simulink model "NeuromuscularModel_3R60_3D"  (R2019b)
settings: Solver=ode15s  StartTime=0.0  StopTime=30  MaxStep=.01  RelTol=1e-4  AbsTol=1e-6  EnableMultiTasking=on
values from neighbouring files (symbols this model uses):
  animFrameRate = 30    [demorun.m]    (also in optimize.m; optimizeCMG.m)
  dt_visual = 1/1000    (= 0.001)    [demorun.m]    (also in evaluateCost.m = 0.0333333333333; optimize.m = 0.0333333333333; optimizeCMG.m = 0.0333333333333; optimize_Conly.m = 0.0333333333333)
  initialTargetAngle = 70*pi/180    (= 1.2217304764)    [setInit.m]
  LPreStimBFSHinit = initConditionsSagittal(12)    [assignInit.m]
  LPreStimGASinit = initConditionsSagittal(13)    [assignInit.m]
  LPreStimGLUinit = initConditionsSagittal(8)    [assignInit.m]
  LPreStimHABinit = initConditionsCoronal(6)    [assignInit.m]
  LPreStimHADinit = initConditionsCoronal(7)    [assignInit.m]
  LPreStimHAMinit = initConditionsSagittal(9)    [assignInit.m]
  LPreStimHFLinit = initConditionsSagittal(7)    [assignInit.m]
  LPreStimRFinit = initConditionsSagittal(10)    [assignInit.m]
  LPreStimSOLinit = initConditionsSagittal(14)    [assignInit.m]
  LPreStimTAinit = initConditionsSagittal(15)    [assignInit.m]
  LPreStimVASinit = initConditionsSagittal(11)    [assignInit.m]
  LTargetAngleInit = initConditionsSagittal(6)    [assignInit.m]
  LTargetAngleRInit = initConditionsCoronal(5)    [assignInit.m]
  N = 133    [vcmaes_1.5cm_0.9ms_Umb10_kneelim1_mstoptorque2.mat]
  RPreStimGLUinit = initConditionsSagittal(18)    [assignInit.m]
  RPreStimHABinit = initConditionsCoronal(9)    [assignInit.m]
  RPreStimHADinit = initConditionsCoronal(10)    [assignInit.m]
  RPreStimHAMinit = initConditionsSagittal(19)    [assignInit.m]
  RPreStimHFLinit = initConditionsSagittal(17)    [assignInit.m]
  RPreStimRFinit = initConditionsSagittal(20)    [assignInit.m]
  RTargetAngleInit = initConditionsSagittal(16)    [assignInit.m]
  RTargetAngleRInit = initConditionsCoronal(8)    [assignInit.m]
undefined symbols (not defined in the file or in its folder): g, GaitState, hatLeftHipToCenterDistWidth, LongDelay, LongLoopDelay, MidDelay, ShortDelay, termination_height, thetaHATref, X, Y, Z
libraries: NeuroMuscularLibrary x105, nesl_utility x22, sm_lib x21, simulink x3, CMGlibrary x1
(part 2 of 3)

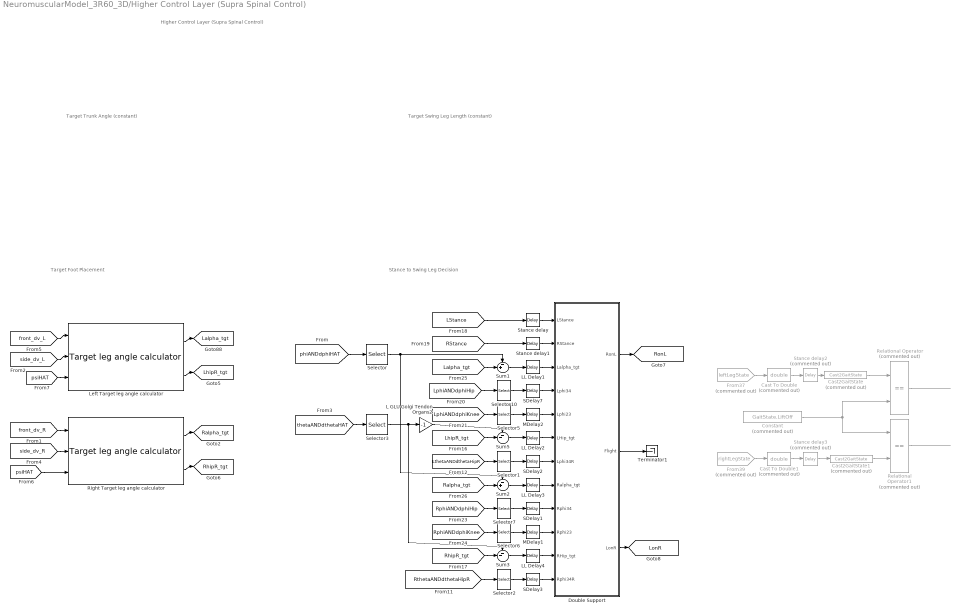
== system NeuromuscularModel_3R60_3D/Higher Control Layer (Supra Spinal Control) ==
  note: Target Foot Placement
  note: Target Swing Leg Length
      | (constant)
  note: Stance to Swing Leg Decision
  note: Target Trunk Angle
      | (constant)
  note: Higher Control Layer
      | (Supra Spinal Control)
  Cast To Double : DataTypeConversion  Commented=on  OutDataTypeStr=double
  Cast To Double1 : DataTypeConversion  Commented=on  OutDataTypeStr=double
  Cast2GaitState : NeuroMuscularLibrary/Cast2GaitState  Commented=on  SystemSampleTime=-1  Latency=0  AutoFrameSizeCalculation=off
  Cast2GaitState1 : NeuroMuscularLibrary/Cast2GaitState  Commented=on  SystemSampleTime=-1  Latency=0  AutoFrameSizeCalculation=off
  Constant : Constant  Commented=on  Value=GaitState.LiftOff
  Double Support : Subsystem
  From37 : From  Commented=on  GotoTag=leftLegState  TagVisibility=global
  From39 : From  Commented=on  GotoTag=rightLegState  TagVisibility=global
  L GLU Golgi Tendon Organs2 : Gain  Gain=-1
  LL Delay1 : TransportDelay  DelayTime=LongLoopDelay/2  InitialOutput=initialTargetAngle
  LL Delay2 : TransportDelay  DelayTime=LongLoopDelay/2
  LL Delay3 : TransportDelay  DelayTime=LongLoopDelay/2  InitialOutput=initialTargetAngle
  LL Delay4 : TransportDelay  DelayTime=LongLoopDelay/2
  Left Target leg angle calculator : NeuroMuscularLibrary/Target leg angle calculator  simbiconLegAngle0=LsimbiconLegAngle0  simbiconGainD=LsimbiconGainD  simbiconGainV=LsimbiconGainV  simbiconLegAngle0_C=LsimbiconLegAngle0_C  simbiconGainD_C=LsimbiconGainD_C  simbiconGainV_C=LsimbiconGainV_C  headingGain=LheadingGain
  MDelay1 : TransportDelay  DelayTime=MidDelay
  MDelay2 : TransportDelay  DelayTime=MidDelay
  Relational Operator : RelationalOperator  Commented=on  Operator===  OutDataTypeStr=boolean  RndMeth=Simplest
  Relational Operator1 : RelationalOperator  Commented=on  Operator===  OutDataTypeStr=boolean  RndMeth=Simplest
  Right Target leg angle calculator : NeuroMuscularLibrary/Target leg angle calculator  simbiconLegAngle0=RsimbiconLegAngle0  simbiconGainD=RsimbiconGainD  simbiconGainV=RsimbiconGainV  simbiconLegAngle0_C=RsimbiconLegAngle0_C  simbiconGainD_C=RsimbiconGainD_C  simbiconGainV_C=RsimbiconGainV_C  headingGain=RheadingGain
  SDelay{1..3,7} (4 alike) : TransportDelay  DelayTime=ShortDelay
  Selector : Selector  InputPortWidth=2  IndexOptions=Index vector (dialog)  Indices=[1]  OutputSizes=1
  Selector{1..2,5..7,10} (6 alike) : Selector  InputPortWidth=2  IndexOptions=Index vector (dialog)  Indices=1  OutputSizes=1
  Selector3 : Selector  InputPortWidth=2  IndexOptions=Index vector (dialog)  Indices=[1]  OutputSizes=1
  Stance delay : TransportDelay  DelayTime=MidDelay
  Stance delay1 : TransportDelay  DelayTime=MidDelay
  Stance delay2 : TransportDelay  Commented=on  DelayTime=MidDelay
  Stance delay3 : TransportDelay  Commented=on  DelayTime=MidDelay
  Sum1 : Sum  Inputs=-+|
  Sum2 : Sum  Inputs=-+|
  Sum3 : Sum  Inputs=--|
  Sum5 : Sum  Inputs=--|
  Terminator1 : Terminator
  tag scope: Lalpha_tgt=global, LhipR_tgt=global, LonR=global, Ralpha_tgt=global, RhipR_tgt=global, RonL=global
  wires:
  [LphiANDdphiHip] -> Selector10/1
  [LphiANDdphiKnee] -> Selector5/1
  Selector10/1 -> SDelay7/1
  Selector5/1 -> MDelay2/1
  [RphiANDdphiHip] -> Selector7/1
  [RphiANDdphiKnee] -> Selector6/1
  Selector7/1 -> SDelay1/1
  Selector6/1 -> MDelay1/1
  Stance delay/1 -> Double Support/1(LStance)
  Stance delay1/1 -> Double Support/2(RStance)
  [LStance] -> Stance delay/1
  [RStance] -> Stance delay1/1
  Double Support/2(Flight) -> Terminator1/1
  LL Delay1/1 -> Double Support/3(Lalpha_tgt)
  LL Delay3/1 -> Double Support/8(Ralpha_tgt)
  SDelay7/1 -> Double Support/4(Lphi34)
  SDelay1/1 -> Double Support/9(Rphi34)
  MDelay2/1 -> Double Support/5(Lphi23)
  MDelay1/1 -> Double Support/10(Rphi23)
  Sum1/1 -> LL Delay1/1
  [Lalpha_tgt] -> Sum1/2
  Selector/1 -> Sum2/1, Sum1/1
  [Ralpha_tgt] -> Sum2/2
  Sum2/1 -> LL Delay3/1
  [LthetaANDdthetaHipR] -> Selector1/1
  Selector1/1 -> SDelay2/1
  SDelay2/1 -> Double Support/7(Lphi34R)
  LL Delay2/1 -> Double Support/6(LHip_tgt)
  Sum5/1 -> LL Delay2/1
  [LhipR_tgt] -> Sum5/2
  Selector3/1 -> L GLU Golgi Tendon Organs2/1, Sum3/1
  L GLU Golgi Tendon Organs2/1 -> Sum5/1
  [RthetaANDdthetaHipR] -> Selector2/1
  Selector2/1 -> SDelay3/1
  SDelay3/1 -> Double Support/12(Rphi34R)
  LL Delay4/1 -> Double Support/11(RHip_tgt)
  Sum3/1 -> LL Delay4/1
  [RhipR_tgt] -> Sum3/2
  [phiANDdphiHAT] -> Selector/1
  [thetaANDdthetaHAT] -> Selector3/1
  Right Target leg angle calculator/2 -> [RhipR_tgt]
  Right Target leg angle calculator/1 -> [Ralpha_tgt]
  Left Target leg angle calculator/2 -> [LhipR_tgt]
  Left Target leg angle calculator/1 -> [Lalpha_tgt]
  [side_dv_R] -> Right Target leg angle calculator/2
  [side_dv_L] -> Left Target leg angle calculator/2
  [front_dv_R] -> Right Target leg angle calculator/1
  [front_dv_L] -> Left Target leg angle calculator/1
  [psiHAT] -> Left Target leg angle calculator/3
  [psiHAT] -> Right Target leg angle calculator/3
  From37/1 -> Cast To Double/1
  Constant/1 -> Relational Operator1/1, Relational Operator/2
  From39/1 -> Cast To Double1/1
  Stance delay3/1 -> Cast2GaitState1/1
  Cast To Double/1 -> Stance delay2/1
  Cast To Double1/1 -> Stance delay3/1
  Cast2GaitState/1 -> Relational Operator/1
  Stance delay2/1 -> Cast2GaitState/1
  Cast2GaitState1/1 -> Relational Operator1/2
  Double Support/1(RonL) -> [RonL]
  Double Support/3(LonR) -> [LonR]
  Relational Operator1/1 -> ?
  Relational Operator/1 -> ?

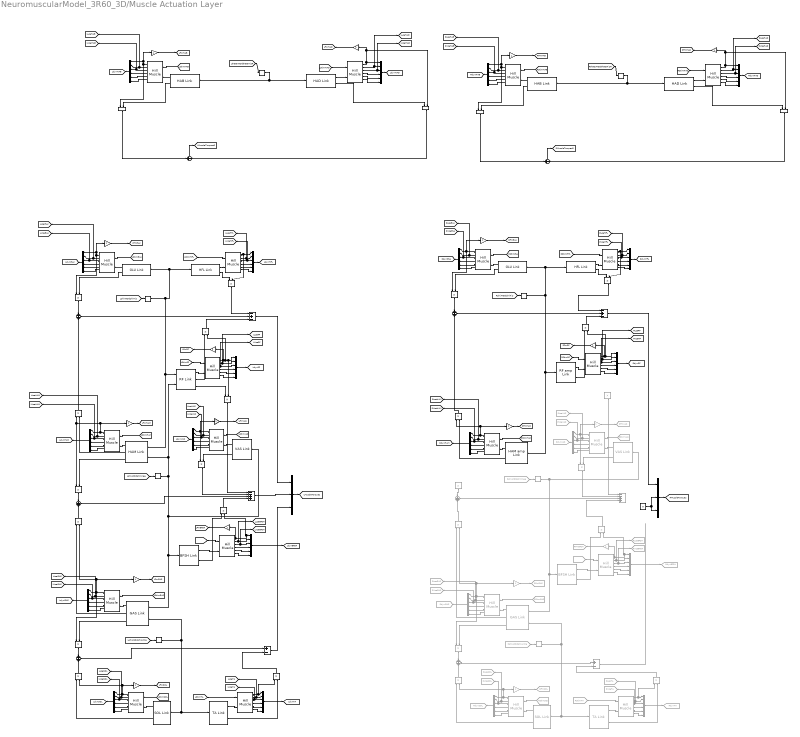
== system NeuromuscularModel_3R60_3D/Muscle Actuation Layer ==
  note: Right Hip Joint
  note: Right Knee Joint
  note: Right Ankle Joint
  note: Left Hip Joint
  note: Left Knee Joint
  note: Left Ankle Joint
  note: Left Leg
  note: Right Leg
  note: Body Mechanics Layer
      | Interface (Left Hip Joint)
  note: Muscle Actuation Layer
      | (Coronal Plane)
  note: Muscle Actuation Layer
      | (Sagittal Plane)
  note: Body Mechanics Layer
      | Interface (Right Hip Joint)
  Add1 : Sum  Inputs=-+-
  Add2 : Sum  Inputs=-+-
  Add3 : Sum  Commented=on  Inputs=--++
  Add4 : Sum  Commented=on  Inputs=+-
  Add5 : Sum  Inputs=--++
  Add6 : Sum  Inputs=+-
  Constant : Constant  Value=0
  From14 : From  Commented=on  GotoTag=RphiANDdphiKnee
  From15 : From  Commented=on  GotoTag=RStimVAS  TagVisibility=global
  From16 : From  Commented=on  GotoTag=RphiANDdphiAnkle  TagVisibility=global
  From17 : From  Commented=on  GotoTag=RStimSOL  TagVisibility=global
  From18 : From  Commented=on  GotoTag=RStimTA  TagVisibility=global
  From19 : From  Commented=on  GotoTag=RStimGAS  TagVisibility=global
  From23 : From  Commented=on  GotoTag=RStimBFSH  TagVisibility=global
  Goto17 : Goto  Commented=on  GotoTag=RFmVAS  TagVisibility=global
  Goto19 : Goto  Commented=on  GotoTag=RFmSOL  TagVisibility=global
  Goto20 : Goto  Commented=on  GotoTag=RLceTA  TagVisibility=global
  Goto21 : Goto  Commented=on  GotoTag=RFmGAS  TagVisibility=global
  Goto31 : Goto  Commented=on  GotoTag=RdynVAS  TagVisibility=global
  Goto32 : Goto  Commented=on  GotoTag=RdynGAS  TagVisibility=global
  Goto33 : Goto  Commented=on  GotoTag=RdynSOL  TagVisibility=global
  Goto34 : Goto  Commented=on  GotoTag=RdynTA  TagVisibility=global
  Goto47 : Goto  Commented=on  GotoTag=RLceVAS  TagVisibility=global
  Goto48 : Goto  Commented=on  GotoTag=RVceVAS  TagVisibility=global
  Goto50 : Goto  Commented=on  GotoTag=RLceGAS  TagVisibility=global
  Goto51 : Goto  Commented=on  GotoTag=RVceGAS  TagVisibility=global
  Goto52 : Goto  Commented=on  GotoTag=RLceSOL  TagVisibility=global
  Goto53 : Goto  Commented=on  GotoTag=RVceSOL  TagVisibility=global
  Goto54 : Goto  Commented=on  GotoTag=RVceTA  TagVisibility=global
  Goto63 : Goto  Commented=on  GotoTag=RdynBFSH  TagVisibility=global
  Goto64 : Goto  Commented=on  GotoTag=RLceBFSH  TagVisibility=global
  Goto65 : Goto  Commented=on  GotoTag=RVceBFSH  TagVisibility=global
  Goto66 : Goto  Commented=on  GotoTag=RFmBFSH  TagVisibility=global
  L  TA Link : NeuroMuscularLibrary/TA Link  SystemSampleTime=-1  Latency=0  AutoFrameSizeCalculation=off
  L BFSH Golgi Tendon Organs : Gain
  L BFSH Link : NeuroMuscularLibrary/BFSH Link  SystemSampleTime=-1  Latency=0  AutoFrameSizeCalculation=off
  L BFSH Muscle : NeuroMuscularLibrary/Hill Muscle  Fmax=FmaxBFSH  lopt=loptBFSH  vmax=vmaxBFSH  lslack=lslackBFSH
  L GAS Golgi Tendon Organs : Gain
  L GAS Link : NeuroMuscularLibrary/GAS Link  SystemSampleTime=-1  Latency=0  AutoFrameSizeCalculation=off
  L GAS Muscle : NeuroMuscularLibrary/Hill Muscle  Fmax=FmaxGAS  lopt=loptGAS  vmax=vmaxGAS  lslack=lslackGAS
  L GLU Golgi Tendon Organs : Gain
  L GLU Link : NeuroMuscularLibrary/GLU Link  SystemSampleTime=-1  Latency=0  AutoFrameSizeCalculation=off
  L GLU Muscle : NeuroMuscularLibrary/Hill Muscle  Fmax=FmaxGLU  lopt=loptGLU  vmax=vmaxGLU  lslack=lslackGLU
  L HAB Golgi Tendon Organs : Gain
  L HAB Link : NeuroMuscularLibrary/HAB Link  SystemSampleTime=-1  Latency=0  AutoFrameSizeCalculation=off
  L HAB Muscle : NeuroMuscularLibrary/Hill Muscle  Fmax=FmaxHAB  lopt=loptHAB  vmax=vmaxHAB  lslack=lslackHAB
  L HAD Golgi Tendon Organs : Gain
  L HAD Link : NeuroMuscularLibrary/HAD Link  SystemSampleTime=-1  Latency=0  AutoFrameSizeCalculation=off
  L HAD Muscle : NeuroMuscularLibrary/Hill Muscle  Fmax=FmaxHAD  lopt=loptHAD  vmax=vmaxHAD  lslack=lslackHAD
  L HAM Golgi Tendon Organs : Gain
  L HAM Link : NeuroMuscularLibrary/HAM Link  SystemSampleTime=-1  Latency=0  AutoFrameSizeCalculation=off
  L HAM Muscle : NeuroMuscularLibrary/Hill Muscle  Fmax=FmaxHAM  lopt=loptHAM  vmax=vmaxHAM  lslack=lslackHAM
  L HFL Link : NeuroMuscularLibrary/HFL Link  SystemSampleTime=-1  Latency=0  AutoFrameSizeCalculation=off
  L HFL Muscle : NeuroMuscularLibrary/Hill Muscle  Fmax=FmaxHFL  lopt=loptHFL  vmax=vmaxHFL  lslack=lslackHFL
  L RF Golgi Tendon Organs : Gain
  L RF Link : NeuroMuscularLibrary/RF Link  SystemSampleTime=-1  Latency=0  AutoFrameSizeCalculation=off
  L RF Muscle : NeuroMuscularLibrary/Hill Muscle  Fmax=FmaxRF  lopt=loptRF  vmax=vmaxRF  lslack=lslackRF
  L SOL Golgi Tendon Organs : Gain
  L SOL Link : NeuroMuscularLibrary/SOL Link  SystemSampleTime=-1  Latency=0  AutoFrameSizeCalculation=off
  L SOL Muscle : NeuroMuscularLibrary/Hill Muscle  Fmax=FmaxSOL  lopt=loptSOL  vmax=vmaxSOL  lslack=lslackSOL
  L TA Muscle : NeuroMuscularLibrary/Hill Muscle  Fmax=FmaxTA  lopt=loptTA  vmax=vmaxTA  lslack=lslackTA
  L VAS Golgi Tendon Organs : Gain
  L VAS Link : NeuroMuscularLibrary/VAS Link  SystemSampleTime=-1  Latency=0  AutoFrameSizeCalculation=off
  L VAS Muscle : NeuroMuscularLibrary/Hill Muscle  Fmax=FmaxVAS  lopt=loptVAS  vmax=vmaxVAS  lslack=lslackVAS
  Mux : Mux  Inputs=3
  Mux1 : Mux  Inputs=3
  Mux{2..10,15..17,19..23} (17 alike) : Mux  Inputs=6
  Mux{11..14,18} (5 alike) : Mux  Commented=on  Inputs=6
  Product{1..2,26..27} (4 alike) : Product  RndMeth=Zero
  R  TA Link : NeuroMuscularLibrary/TA Link  Commented=on  SystemSampleTime=-1  Latency=0  AutoFrameSizeCalculation=off
  R BFSH Golgi Tendon Organs : Gain  Commented=on
  R BFSH Link : NeuroMuscularLibrary/BFSH Link  Commented=on  SystemSampleTime=-1  Latency=0  AutoFrameSizeCalculation=off
  R BFSH Muscle : NeuroMuscularLibrary/Hill Muscle  Commented=on  Fmax=FmaxBFSH  lopt=loptBFSH  vmax=vmaxBFSH  lslack=lslackBFSH
  R GAS Golgi Tendon Organs : Gain  Commented=on
  R GAS Link : NeuroMuscularLibrary/GAS Link  Commented=on  SystemSampleTime=-1  Latency=0  AutoFrameSizeCalculation=off
  R GAS Muscle : NeuroMuscularLibrary/Hill Muscle  Commented=on  Fmax=FmaxGAS  lopt=loptGAS  vmax=vmaxGAS  lslack=lslackGAS
  R GLU Golgi Tendon Organs : Gain
  R GLU Link : NeuroMuscularLibrary/GLU Link  SystemSampleTime=-1  Latency=0  AutoFrameSizeCalculation=off
  R GLU amp Muscle : NeuroMuscularLibrary/Hill Muscle  Fmax=FmaxGLUamp  lopt=loptGLUamp  vmax=vmaxGLUamp  lslack=lslackGLUamp
  R HAB Golgi Tendon Organs : Gain
  R HAB Link : NeuroMuscularLibrary/HAB Link  SystemSampleTime=-1  Latency=0  AutoFrameSizeCalculation=off
  R HAB amp Muscle : NeuroMuscularLibrary/Hill Muscle  Fmax=FmaxHABamp  lopt=loptHABamp  vmax=vmaxHABamp  lslack=lslackHABamp
  R HAD Golgi Tendon Organs : Gain
  R HAD Link : NeuroMuscularLibrary/HAD Link  SystemSampleTime=-1  Latency=0  AutoFrameSizeCalculation=off
  R HAD Muscle : NeuroMuscularLibrary/Hill Muscle  Fmax=FmaxHADamp  lopt=loptHADamp  vmax=vmaxHADamp  lslack=lslackHADamp
  R HAM Golgi Tendon Organs : Gain
  R HAM amp Link : NeuroMuscularLibrary/HAM amp Link  SystemSampleTime=-1  Latency=0  AutoFrameSizeCalculation=off
  R HAM amp Muscle : NeuroMuscularLibrary/Hill Muscle  Fmax=FmaxHAMamp  lopt=loptHAMamp  vmax=vmaxHAMamp  lslack=lslackHAMamp
  R HFL  Link : NeuroMuscularLibrary/HFL Link  SystemSampleTime=-1  Latency=0  AutoFrameSizeCalculation=off
  R HFL amp Muscle : NeuroMuscularLibrary/Hill Muscle  Fmax=FmaxHFLamp  lopt=loptHFLamp  vmax=vmaxHFLamp  lslack=lslackHFLamp
  R RF Golgi Tendon Organs : Gain
  R RF amp Link : NeuroMuscularLibrary/RF amp Link  SystemSampleTime=-1  Latency=0  AutoFrameSizeCalculation=off
  R RF amp Muscle : NeuroMuscularLibrary/Hill Muscle  Fmax=FmaxRFamp  lopt=loptRFamp  vmax=vmaxRFamp  lslack=lslackRFamp
  R SOL Golgi Tendon Organs : Gain  Commented=on
  R SOL Link : NeuroMuscularLibrary/SOL Link  Commented=on  SystemSampleTime=-1  Latency=0  AutoFrameSizeCalculation=off
  R SOL Muscle : NeuroMuscularLibrary/Hill Muscle  Commented=on  Fmax=FmaxSOL  lopt=loptSOL  vmax=vmaxSOL  lslack=lslackSOL
  R TA Muscle : NeuroMuscularLibrary/Hill Muscle  Commented=on  Fmax=FmaxTA  lopt=loptTA  vmax=vmaxTA  lslack=lslackTA
  R VAS Golgi Tendon Organs : Gain  Commented=on
  R VAS Link : NeuroMuscularLibrary/VAS Link  Commented=on  SystemSampleTime=-1  Latency=0  AutoFrameSizeCalculation=off
  R VAS Muscle : NeuroMuscularLibrary/Hill Muscle  Commented=on  Fmax=FmaxVAS  lopt=loptVAS  vmax=vmaxVAS  lslack=lslackVAS
  Selector{1,4..8} (6 alike) : Selector  InputPortWidth=2  IndexOptions=Index vector (dialog)  Indices=1  OutputSizes=1
  Selector2 : Selector  Commented=on  InputPortWidth=2  IndexOptions=Index vector (dialog)  Indices=1  OutputSizes=1
  Selector3 : Selector  Commented=on  InputPortWidth=2  IndexOptions=Index vector (dialog)  Indices=1  OutputSizes=1
  Sum{1,3..4,8} (4 alike) : Sum  Inputs=+|+
  Sum11 : Sum  Commented=on  Inputs=+|+
  Sum15 : Sum  Commented=on  Inputs=+|+
  Sum2 : Sum  Inputs=+-
  Sum25 : Sum  Inputs=+-
  tau = r*F{1..11,18..21,24} (16 alike) : Product
  tau = r*F{12..17,22..23} (8 alike) : Product  Commented=on
  tag scope: LFmBFSH=global, LFmGAS=global, LFmGLU=global, LFmHAB=global, LFmHAD=global, LFmHAM=global, LFmRF=global, LFmSOL=global, LFmVAS=global, LLceBFSH=global, LLceGAS=global, LLceGLU=global, LLceHAB=global, LLceHAD=global, LLceHAM=global, LLceHFL=global, LLceRF=global, LLceSOL=global, LLceTA=global, LLceVAS=global, LMuscleTorques=global, LMuscleTorquesR=global, LVceBFSH=global, LVceGAS=global, LVceGLU=global, LVceHAB=global, LVceHAD=global, LVceHAM=global, LVceHFL=global, LVceRF=global, LVceSOL=global, LVceTA=global, LVceVAS=global, LdynBFSH=global, LdynGAS=global, LdynGLU=global, LdynHAB=global, LdynHAD=global, LdynHAM=global, LdynHFL=global, LdynRF=global, LdynSOL=global, LdynTA=global, LdynVAS=global, RFmGLU=global, RFmHAB=global, RFmHAD=global, RFmHAM=global, RFmRF=global, RLceGLU=global, RLceHAB=global, RLceHAD=global, RLceHAM=global, RLceHFL=global, RLceRF=global, RMuscleTorques=global, RMuscleTorquesR=global, RVceGLU=global, RVceHAB=global, RVceHAD=global, RVceHAM=global, RVceHFL=global, RVceRF=global, RdynGLU=global, RdynHAB=global, RdynHAD=global, RdynHAM=global, RdynHFL=global, RdynRF=global
  wires:
  R HAM amp Link/1 -> R HAM amp Muscle/2
  R HAM amp Link/2 -> tau = r*F9/2
  R HAM amp Muscle/5 -> Mux7/5
  Mux7/1 -> [RdynHAM]
  R HAM amp Muscle/3 -> [RVceHAM], Mux7/3
  R HAM amp Muscle/4 -> Mux7/4
  [RphiANDdphiHip] -> Selector1/1
  Selector1/1 -> R HAM amp Link/1, R RF amp Link/1, R GLU Link/1, R HFL  Link/1
  Add2/1 -> Mux/1
  R GLU Link/1 -> R GLU amp Muscle/2
  [RStimGLU] -> R GLU amp Muscle/1
  R GLU amp Muscle/5 -> Mux9/5
  R GLU amp Muscle/2 -> [RLceGLU], Mux9/2
  R GLU amp Muscle/3 -> [RVceGLU], Mux9/3
  R GLU amp Muscle/4 -> Mux9/4
  R GLU Link/2 -> tau = r*F10/2
  R GLU amp Muscle/1 -> Mux9/1, R GLU Golgi Tendon Organs/1, tau = r*F10/1
  R GLU Golgi Tendon Organs/1 -> [RFmGLU]
  R HFL  Link/1 -> R HFL amp Muscle/2
  [RStimHFL] -> R HFL amp Muscle/1
  R HFL amp Muscle/5 -> Mux10/5
  Mux10/1 -> [RdynHFL]
  R HFL amp Muscle/4 -> Mux10/4
  R HFL amp Muscle/3 -> [RVceHFL], Mux10/3
  R HFL  Link/2 -> tau = r*F11/1
  R HFL amp Muscle/1 -> Mux10/1, tau = r*F11/2
  R HAM Golgi Tendon Organs/1 -> [RFmHAM]
  [RStimHAM] -> R HAM amp Muscle/1
  R VAS Link/1 -> R VAS Muscle/2
  R VAS Muscle/5 -> Mux11/5
  Mux11/1 -> Goto31/1
  R VAS Muscle/2 -> Goto47/1, Mux11/2
  R VAS Muscle/3 -> Goto48/1, Mux11/3
  R VAS Muscle/4 -> Mux11/4
  R VAS Muscle/1 -> R VAS Golgi Tendon Organs/1, Mux11/1, tau = r*F13/1
  R VAS Golgi Tendon Organs/1 -> Goto17/1
  R VAS Link/2 -> tau = r*F13/2
  Sum11/1 -> Add3/3  "Knee Flexion Torque"
  From15/1 -> R VAS Muscle/1
  From14/1 -> Selector3/1
  R SOL Muscle/1 -> R SOL Golgi Tendon Organs/1, tau = r*F12/2, Mux13/1
  R SOL Muscle/5 -> Mux13/5
  Mux13/1 -> Goto33/1
  R SOL Muscle/2 -> Goto52/1, Mux13/2
  R SOL Muscle/3 -> Goto53/1, Mux13/3
  R SOL Muscle/4 -> Mux13/4
  R SOL Link/2 -> tau = r*F12/1
  R SOL Link/1 -> R SOL Muscle/2
  R SOL Golgi Tendon Organs/1 -> Goto19/1
  From17/1 -> R SOL Muscle/1
  Selector2/1 -> R GAS Link/2, R  TA Link/1, R SOL Link/1
  From16/1 -> Selector2/1
  Add4/1 -> ?
  R  TA Link/1 -> R TA Muscle/2
  R TA Muscle/1 -> tau = r*F15/1, Mux14/1
  R TA Muscle/5 -> Mux14/5
  Mux14/1 -> Goto34/1
  R TA Muscle/4 -> Mux14/4
  R TA Muscle/3 -> Mux14/3, Goto54/1
  From18/1 -> R TA Muscle/1
  R  TA Link/2 -> tau = r*F15/2
  tau = r*F15/1 -> Add4/2
  R GAS Link/1 -> R GAS Muscle/2
  Selector3/1 -> R VAS Link/1, R GAS Link/1, R BFSH Link/1
  R GAS Muscle/5 -> Mux12/5
  Mux12/1 -> Goto32/1
  R GAS Muscle/2 -> Goto50/1, Mux12/2
  R GAS Muscle/3 -> Goto51/1, Mux12/3
  R GAS Muscle/4 -> Mux12/4
  R GAS Link/2 -> tau = r*F16/1
  From19/1 -> R GAS Muscle/1
  tau = r*F12/1 -> Sum15/2
  Sum15/1 -> Add4/1
  R GAS Link/3 -> tau = r*F17/2
  tau = r*F17/1 -> Sum15/1
  R GAS Muscle/1 -> Mux12/1, tau = r*F16/2, R GAS Golgi Tendon Organs/1, tau = r*F17/1
  R GAS Golgi Tendon Organs/1 -> Goto21/1
  tau = r*F9/1 -> Sum8/2  "HAM"
  tau = r*F10/1 -> Sum8/1  "GLU"
  tau = r*F11/1 -> Add2/1  "HFL"
  R HAM amp Muscle/1 -> tau = r*F9/1, R HAM Golgi Tendon Organs/1, Mux7/1
  Sum8/1 -> Add2/2  "Hip Extension Moment"
  tau = r*F16/1 -> Sum11/2  "GAS"
  tau = r*F14/1 -> Sum11/1  "HAM"
  tau = r*F13/1 -> Add3/2  "VAS"
  R TA Muscle/2 -> Goto20/1, Mux14/2
  Mux9/1 -> [RdynGLU]
  Mux/1 -> [RMuscleTorques]
  L HAM Link/1 -> L HAM Muscle/2
  L HAM Link/2 -> tau = r*F18/2
  L HAM Muscle/5 -> Mux8/5
  Mux8/1 -> [LdynHAM]
  L HAM Muscle/3 -> [LVceHAM], Mux8/3
  L HAM Muscle/4 -> Mux8/4
  [LphiANDdphiHip] -> Selector4/1
  Selector4/1 -> L GLU Link/1, L HFL Link/1, L RF Link/1, L HAM Link/1
  Add1/1 -> Mux1/1
  L GLU Link/1 -> L GLU Muscle/2
  [LStimGLU] -> L GLU Muscle/1
  L GLU Muscle/5 -> Mux15/5
  L GLU Muscle/2 -> Mux15/2, [LLceGLU]
  L GLU Muscle/3 -> Mux15/3, [LVceGLU]
  L GLU Muscle/4 -> Mux15/4
  L GLU Link/2 -> tau = r*F1/2
  L GLU Muscle/1 -> Mux15/1, L GLU Golgi Tendon Organs/1, tau = r*F1/1
  L GLU Golgi Tendon Organs/1 -> [LFmGLU]
  L HFL Link/1 -> L HFL Muscle/2
  [LStimHFL] -> L HFL Muscle/1
  L HFL Muscle/5 -> Mux2/5
  Mux2/1 -> [LdynHFL]
  L HFL Muscle/4 -> Mux2/4
  L HFL Muscle/3 -> [LVceHFL], Mux2/3
  L HFL Link/2 -> tau = r*F2/1
  L HFL Muscle/1 -> Mux2/1, tau = r*F2/2
  L HAM Golgi Tendon Organs/1 -> [LFmHAM]
  [LStimHAM] -> L HAM Muscle/1
  L VAS Link/1 -> L VAS Muscle/2
  L VAS Muscle/5 -> Mux3/5
  Mux3/1 -> [LdynVAS]
  L VAS Muscle/2 -> [LLceVAS], Mux3/2
  L VAS Muscle/3 -> [LVceVAS], Mux3/3
  L VAS Muscle/4 -> Mux3/4
  L VAS Muscle/1 -> L VAS Golgi Tendon Organs/1, Mux3/1, tau = r*F4/1
  L VAS Golgi Tendon Organs/1 -> [LFmVAS]
  L VAS Link/2 -> tau = r*F4/2
  L HAM Link/3 -> tau = r*F5/2
  Sum1/1 -> Add5/3  "Knee Flexion Torque"
  [LStimVAS] -> L VAS Muscle/1
  [LphiANDdphiKnee] -> Selector6/1
  L SOL Muscle/1 -> L SOL Golgi Tendon Organs/1, tau = r*F3/2, Mux5/1
  L SOL Muscle/5 -> Mux5/5
  Mux5/1 -> [LdynSOL]
  L SOL Muscle/3 -> [LVceSOL], Mux5/3
  L SOL Muscle/4 -> Mux5/4
  L SOL Link/2 -> tau = r*F3/1
  L SOL Link/1 -> L SOL Muscle/2
  L SOL Golgi Tendon Organs/1 -> [LFmSOL]
  [LStimSOL] -> L SOL Muscle/1
  Selector5/1 -> L GAS Link/2, L  TA Link/1, L SOL Link/1
  [LphiANDdphiAnkle] -> Selector5/1
  Add6/1 -> Mux1/3
  L  TA Link/1 -> L TA Muscle/2
  L TA Muscle/1 -> tau = r*F6/1, Mux6/1
  L TA Muscle/5 -> Mux6/5
  Mux6/1 -> [LdynTA]
  L TA Muscle/4 -> Mux6/4
  L TA Muscle/3 -> Mux6/3, [LVceTA]
  [LStimTA] -> L TA Muscle/1
  L  TA Link/2 -> tau = r*F6/2
  tau = r*F6/1 -> Add6/2
  L GAS Link/1 -> L GAS Muscle/2
  Selector6/1 -> L GAS Link/1, L BFSH Link/1, L VAS Link/1, L RF Link/2, L HAM Link/2
  L GAS Muscle/5 -> Mux4/5
  Mux4/1 -> [LdynGAS]
  L GAS Muscle/2 -> [LLceGAS], Mux4/2
  L GAS Muscle/3 -> [LVceGAS], Mux4/3
  L GAS Muscle/4 -> Mux4/4
  L GAS Link/2 -> tau = r*F7/1
  [LStimGAS] -> L GAS Muscle/1
  tau = r*F3/1 -> Sum3/2
  Sum3/1 -> Add6/1
  L GAS Link/3 -> tau = r*F8/2
  tau = r*F8/1 -> Sum3/1
  L GAS Muscle/1 -> Mux4/1, tau = r*F7/2, L GAS Golgi Tendon Organs/1, tau = r*F8/1
  L GAS Golgi Tendon Organs/1 -> [LFmGAS]
  tau = r*F18/1 -> Sum4/2  "HAM"
  tau = r*F1/1 -> Sum4/1  "GLU"
  tau = r*F2/1 -> Add1/1  "HFL"
  L HAM Muscle/1 -> tau = r*F5/1, tau = r*F18/1, L HAM Golgi Tendon Organs/1, Mux8/1
  Sum4/1 -> Add1/2  "Hip Extension Moment"
  tau = r*F7/1 -> Sum1/2  "GAS"
  tau = r*F5/1 -> Sum1/1  "HAM"
  tau = r*F4/1 -> Add5/2  "VAS"
  L TA Muscle/2 -> [LLceTA], Mux6/2
  Mux15/1 -> [LdynGLU]
  Mux1/1 -> [LMuscleTorques]
  L GLU Muscle/6 -> Mux15/6
  L HFL Muscle/6 -> Mux2/6
  L HAM Muscle/6 -> Mux8/6
  L VAS Muscle/6 -> Mux3/6
  L GAS Muscle/6 -> Mux4/6
  L SOL Muscle/6 -> Mux5/6
  L TA Muscle/6 -> Mux6/6
  R SOL Muscle/6 -> Mux13/6
  R TA Muscle/6 -> Mux14/6
  R GAS Muscle/6 -> Mux12/6
  R HAM amp Muscle/6 -> Mux7/6
  R VAS Muscle/6 -> Mux11/6
  R HFL amp Muscle/6 -> Mux10/6
  R GLU amp Muscle/6 -> Mux9/6
  R HFL amp Muscle/2 -> [RLceHFL], Mux10/2
  R HAM amp Muscle/2 -> [RLceHAM], Mux7/2
  L HFL Muscle/2 -> [LLceHFL], Mux2/2
  L HAM Muscle/2 -> [LLceHAM], Mux8/2
  L SOL Muscle/2 -> [LLceSOL], Mux5/2
  L BFSH Muscle/3 -> [LVceBFSH], Mux16/3
  [LStimBFSH] -> L BFSH Muscle/1
  L BFSH Link/2 -> tau = r*F19/1
  L BFSH Golgi Tendon Organs/1 -> [LFmBFSH]
  L BFSH Muscle/6 -> Mux16/6
  L BFSH Muscle/4 -> Mux16/4
  L BFSH Link/1 -> L BFSH Muscle/2
  Mux16/1 -> [LdynBFSH]
  L BFSH Muscle/2 -> [LLceBFSH], Mux16/2
  L BFSH Muscle/5 -> Mux16/5
  L BFSH Muscle/1 -> tau = r*F19/2, Mux16/1, L BFSH Golgi Tendon Organs/1
  tau = r*F19/1 -> Add5/4  "BFSH"
  L RF Muscle/3 -> [LVceRF], Mux17/3
  [LStimRF] -> L RF Muscle/1
  L RF Link/3 -> tau = r*F20/2
  L RF Golgi Tendon Organs/1 -> [LFmRF]
  L RF Muscle/6 -> Mux17/6
  L RF Muscle/4 -> Mux17/4
  L RF Link/1 -> L RF Muscle/2
  Mux17/1 -> [LdynRF]
  L RF Muscle/2 -> [LLceRF], Mux17/2
  L RF Muscle/5 -> Mux17/5
  L RF Muscle/1 -> tau = r*F21/2, Mux17/1, tau = r*F20/1, L RF Golgi Tendon Organs/1
  L RF Link/2 -> tau = r*F21/1
  tau = r*F21/1 -> Add1/3  "RF"
  tau = r*F20/1 -> Add5/1  "RF"
  R BFSH Muscle/3 -> Goto65/1, Mux18/3
  From23/1 -> R BFSH Muscle/1
  R BFSH Muscle/1 -> tau = r*F22/2, Mux18/1, R BFSH Golgi Tendon Organs/1
  R BFSH Muscle/4 -> Mux18/4
  R BFSH Golgi Tendon Organs/1 -> Goto66/1
  R BFSH Muscle/5 -> Mux18/5
  Mux18/1 -> Goto63/1
  R BFSH Muscle/2 -> Goto64/1, Mux18/2
  R BFSH Link/1 -> R BFSH Muscle/2
  R BFSH Link/2 -> tau = r*F22/1
  R BFSH Muscle/6 -> Mux18/6
  tau = r*F22/1 -> Add3/4  "BFSH"
  [RStimRF] -> R RF amp Muscle/1
  R RF amp Muscle/3 -> [RVceRF], Mux19/3
  R RF amp Muscle/4 -> Mux19/4
  R RF amp Muscle/6 -> Mux19/6
  R RF amp Muscle/5 -> Mux19/5
  R RF amp Muscle/2 -> [RLceRF], Mux19/2
  R RF amp Muscle/1 -> tau = r*F24/2, Mux19/1, R RF Golgi Tendon Organs/1
  Mux19/1 -> [RdynRF]
  R RF amp Link/2 -> tau = r*F24/1
  R RF Golgi Tendon Organs/1 -> [RFmRF]
  R RF amp Link/1 -> R RF amp Muscle/2
  tau = r*F24/1 -> Add2/3  "RF"
  tau = r*F23/1 -> Add3/1  "RF"
  Product27/1 -> Sum25/2
  L HAD Link/2 -> Product27/1
  Selector7/1 -> L HAB Link/1, L HAD Link/1
  Product26/1 -> Sum25/1
  L HAB Muscle/6 -> Mux20/6
  L HAB Muscle/1 -> Product26/1, Mux20/1, L HAB Golgi Tendon Organs/1
  L HAB Golgi Tendon Organs/1 -> [LFmHAB]
  L HAB Muscle/4 -> Mux20/4
  L HAB Muscle/2 -> Mux20/2, [LLceHAB]
  L HAB Muscle/5 -> Mux20/5
  L HAB Link/1 -> L HAB Muscle/2
  L HAB Link/2 -> Product26/2
  L HAB Muscle/3 -> Mux20/3, [LVceHAB]
  [LStimHAB] -> L HAB Muscle/1
  Mux20/1 -> [LdynHAB]
  [LthetaANDdthetaHipR] -> Selector7/1
  L HAD Link/1 -> L HAD Muscle/2
  [LStimHAD] -> L HAD Muscle/1
  L HAD Golgi Tendon Organs/1 -> [LFmHAD]
  L HAD Muscle/2 -> Mux21/2, [LLceHAD]
  L HAD Muscle/1 -> Mux21/1, Product27/2, L HAD Golgi Tendon Organs/1
  L HAD Muscle/3 -> [LVceHAD], Mux21/3
  L HAD Muscle/4 -> Mux21/4
  L HAD Muscle/5 -> Mux21/5
  L HAD Muscle/6 -> Mux21/6
  Mux21/1 -> [LdynHAD]
  Sum25/1 -> [LMuscleTorquesR]
  R HAD Muscle/6 -> Mux23/6
  Selector8/1 -> R HAB Link/1, R HAD Link/1
  R HAD Link/2 -> Product2/1
  R HAD Golgi Tendon Organs/1 -> [RFmHAD]
  [RStimHAD] -> R HAD Muscle/1
  Mux23/1 -> [RdynHAD]
  Sum2/1 -> [RMuscleTorquesR]
  Mux22/1 -> [RdynHAB]
  R HAB Golgi Tendon Organs/1 -> [RFmHAB]
  Product1/1 -> Sum2/1
  Product2/1 -> Sum2/2
  R HAD Muscle/5 -> Mux23/5
  R HAD Muscle/2 -> Mux23/2, [RLceHAD]
  R HAD Muscle/3 -> [RVceHAD], Mux23/3
  R HAD Link/1 -> R HAD Muscle/2
  [RthetaANDdthetaHipR] -> Selector8/1
  R HAD Muscle/1 -> Mux23/1, Product2/2, R HAD Golgi Tendon Organs/1
  R HAB Link/2 -> Product1/2
  R HAB amp Muscle/5 -> Mux22/5
  R HAB amp Muscle/2 -> Mux22/2, [RLceHAB]
  R HAD Muscle/4 -> Mux23/4
  R HAB Link/1 -> R HAB amp Muscle/2
  R HAB amp Muscle/4 -> Mux22/4
  R HAB amp Muscle/3 -> Mux22/3, [RVceHAB]
  R HAB amp Muscle/6 -> Mux22/6
  R HAB amp Muscle/1 -> Product1/1, Mux22/1, R HAB Golgi Tendon Organs/1
  [RStimHAB] -> R HAB amp Muscle/1
  Add5/1 -> Mux1/2
  Constant/1 -> Mux/3, Mux/2
